simulink model "power_transfo"  (Simulink 6.0)
settings: Solver=ode15s  SolverMode=SingleTasking  StartTime=0.0  StopTime=0.2  RelTol=1e-3  AbsTol=1e-6
libraries: powerlib x13, powerlib_extras x1
settings Model: Creator=patrice  LastModifiedBy=batserve  ExtModeTrigMode=oneshot  ExtModeArmWhenConnect=off  ExtModeAutoUpdateStatusClock=off
settings DataIOCC: LimitDataPoints=off  SignalLoggingName=sigsOut
settings OptimizationCC: BlockReduction=off  BooleanDataType=off
settings DebuggingCC: CheckExecutionContextPreStartOutputMsg=on  CheckExecutionContextRuntimeOutputMsg=on  SolverPrmCheckMsg=none
settings HardwareCC: TargetUnknown=on
settings RTWCC: TemplateMakefile=grt_unix.tmf

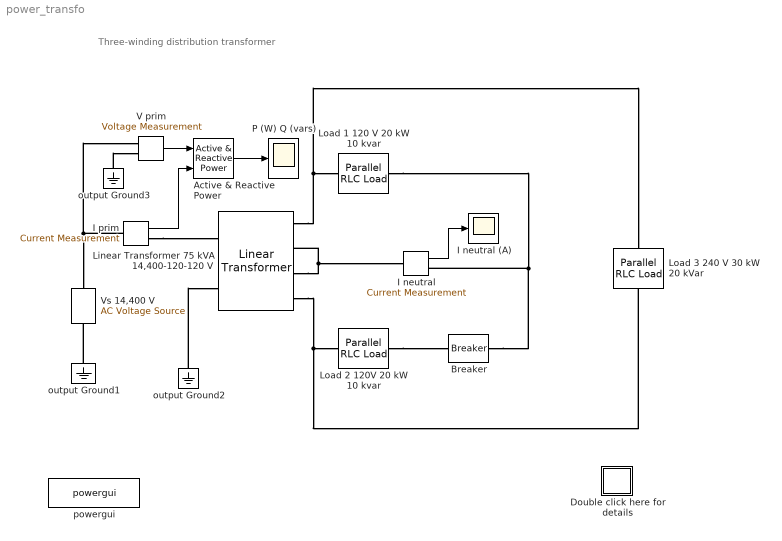
== system power_transfo ==
  note: Three-winding distribution transformer
  Active & Reactive Power : powerlib_extras/Measurements/Active & Reactive Power  f1=60
  Breaker : powerlib/Elements/Breaker  BreakerResistance=1e-5  InitialState=1  SnubberResistance=inf  SnubberCapacitance=0  SwitchingTimes=[ .05 ]  External=off  Measurements=None
      settings: AttributesFormatString=\n
  Double click here for details : Subsystem
      mask Display: disp('?')
  I neutral : powerlib/Measurements/Current Measurement  Tag=PoWeRsYsTeMmEaSuReMeNt  PhasorSimulation=off  OutputType=Magnitude  PSBequivalent=0
  I neutral (A) : Scope
      settings: TickLabels=on  TimeRange=0.2  YMin=-300  YMax=300  DataFormat=Array
  I prim : powerlib/Measurements/Current Measurement  Tag=PoWeRsYsTeMmEaSuReMeNt  PhasorSimulation=off  OutputType=Magnitude  PSBequivalent=0
  Linear Transformer 75 kVA 14,400-120-120 V : powerlib/Elements/Linear Transformer  PhysicalDomain=powersysdomain  SubClassName=unknown  LeftPortType=p1  RightPortType=p1  LConnTagsString=a|b  RConnTagsString=A|B|C|D  NominalPower=[75e3,60]  winding1=[14.4e3 0.01,0.03]  winding2=[120,0.02,0]  ThreeWindings=on  winding3=[120,0.02,0]  RmLm=[50,50]  Measurements=None
  Load 1 120 V 20 kW 10 kvar : powerlib/Elements/Parallel RLC Load  PhysicalDomain=powersysdomain  SubClassName=unknown  LeftPortType=p1  RightPortType=p1  LConnTagsString=a  RConnTagsString=__new0  NominalVoltage=120  NominalFrequency=60  ActivePower=20e3  InductivePower=10e3  CapacitivePower=0  Measurements=None
      settings: AttributesFormatString=\n
  Load 2 120V 20 kW 10 kvar : powerlib/Elements/Parallel RLC Load  PhysicalDomain=powersysdomain  SubClassName=unknown  LeftPortType=p1  RightPortType=p1  LConnTagsString=a  RConnTagsString=__new0  NominalVoltage=120  NominalFrequency=60  ActivePower=20e3  InductivePower=10e3  CapacitivePower=0  Measurements=None
      settings: AttributesFormatString=\n
  Load 3 240 V 30 kW  20 kVar : powerlib/Elements/Parallel RLC Load  Orientation=down  PhysicalDomain=powersysdomain  SubClassName=unknown  LeftPortType=p1  RightPortType=p1  LConnTagsString=a  RConnTagsString=__new0  NominalVoltage=240  NominalFrequency=60  ActivePower=30e3  InductivePower=0  CapacitivePower=20e3  Measurements=None
      settings: AttributesFormatString=\n
  P (W) Q (vars) : Scope
      settings: TickLabels=on  TimeRange=0.2  YMin=-20000  YMax=80000  DataFormat=Array
  V prim : powerlib/Measurements/Voltage Measurement  Tag=PoWeRsYsTeMmEaSuReMeNt  PhasorSimulation=off  OutputType=Magnitude  PSBequivalent=0
  Vs 14,400 V : powerlib/Electrical Sources/AC Voltage Source  Description=source block  Orientation=up  Amplitude=14400*sqrt(2)  Phase=0  Frequency=60  SampleTime=0  Measurements=None
      settings: AttributesFormatString=\n
  output Ground1 : powerlib/Elements/Ground  Orientation=down  PhysicalDomain=powersysdomain  SubClassName=unknown  LeftPortType=p1  RightPortType=p1  LConnTagsString=a
  output Ground2 : powerlib/Elements/Ground  Orientation=down  PhysicalDomain=powersysdomain  SubClassName=unknown  LeftPortType=p1  RightPortType=p1  LConnTagsString=a
  output Ground3 : powerlib/Elements/Ground  Orientation=down  PhysicalDomain=powersysdomain  SubClassName=unknown  LeftPortType=p1  RightPortType=p1  LConnTagsString=a
  powergui : powerlib/powergui  Priority=2  Frange=logspace(0,3,50)  Ylog=off  Xlog=off  save=off  variable=ZData  ZoomFFT=on  StartTime=0.0  cycles=1  DisplayStyle=off  fundamental=60  FreqAxis=off  MaxFrequency=1000  frequencyindice=1  frequencyindicesteady=1  RmsSteady=1  display=off  Ts=0  methode=off  frequency=60  echomessages=on
  wires:
  I prim/1 -> Active & Reactive Power/2
  V prim/1 -> Active & Reactive Power/1
  I neutral/1 -> I neutral (A)/1
  Active & Reactive Power/1 -> P (W) Q (vars)/1
  connections:
  output Ground1/LConn1 -- Vs 14,400 V/LConn1
  I prim/RConn1 -- Linear Transformer 75 kVA 14,400-120-120 V/LConn1
  output Ground2/LConn1 -- Linear Transformer 75 kVA 14,400-120-120 V/LConn2
  I prim/LConn1 -- Vs 14,400 V/RConn1 -- V prim/LConn1
  output Ground3/LConn1 -- V prim/LConn2
  Linear Transformer 75 kVA 14,400-120-120 V/RConn1 -- Load 3 240 V 30 kW  20 kVar/LConn1 -- Load 1 120 V 20 kW 10 kvar/LConn1
  Load 1 120 V 20 kW 10 kvar/RConn1 -- I neutral/RConn1 -- Breaker/RConn1
  Load 3 240 V 30 kW  20 kVar/RConn1 -- Linear Transformer 75 kVA 14,400-120-120 V/RConn4 -- Load 2 120V 20 kW 10 kvar/LConn1
  Load 2 120V 20 kW 10 kvar/RConn1 -- Breaker/LConn1
  Linear Transformer 75 kVA 14,400-120-120 V/RConn3 -- Linear Transformer 75 kVA 14,400-120-120 V/RConn2 -- I neutral/LConn1

== system power_transfo/Double click here for details ==
  note: This demonstration illustrates the  use of the linear transformer to simulate
      | a  three-winding distribution transformer rated 75 kVA - 14400/120/120 V.
  note: The transformer primary is connected to a high voltage source (14,400 V rms).
      | Two identical inductive loads (20 kW -10 kvar) are connected to the two secondaries.
      | A third capacitive load (30 kW -20 kvar) is fed at 240 V.
      |
      | Initially, the circuit breaker in series with Load 2 is closed, so that the system is balanced.
  note: Open the powergui block to obtain the initial voltage and current phasors in steady state.
      | As loads are balanced the neutral current is practically zero.
      |
      | Furthermore, as the inductive reactive power of Load 1 and Load 2 (2*10 kvar) is compensated by the capacitive reactive power
      | of Load 3 (20 kvar), the primary current is almost in phase with voltage  The small phase shift (-2.8deg.) is due to
      | the  reactive power associated with transformer reactive losses.
      |
      | Open the two scopes and start the simulation. The following observations can be made:
      |
      | When the circuit breaker opens, a current starts to  flow in the neutral as a result of the load unbalance.
      | The active power computed from the primary voltage and current is measured by a Simulink block which can be found
      | in the Extras/Measurement library. When the breaker opens, the active power decreases from 70 kW to 50 kW.
  note: Circuit Description
  note: Demonstration
  note: G. Sybille (Hydro-Quebec)
